simulink model "TAMC_PMSM"  (R2016b)
settings: Solver=ode15s  StartTime=0.0  StopTime=0.6  RelTol=1e-4
InitFcn:
  | Ts=10e-6;
  | R=0.958;
  | Ld=5.25e-3;
  | Lq=12e-3;
  | Pn=4;
  | flux=0.1827;
undefined symbols (not defined in the file or in its folder): DiscIntNeverNeededParam
libraries: powerlib x33, powerlib_extras x2
settings Model: Creator=ChenNingke  LastModifiedBy=CNK
settings SolverCC: MaxConsecutiveZCs=100000  ZeroCrossAlgorithm=Adaptive

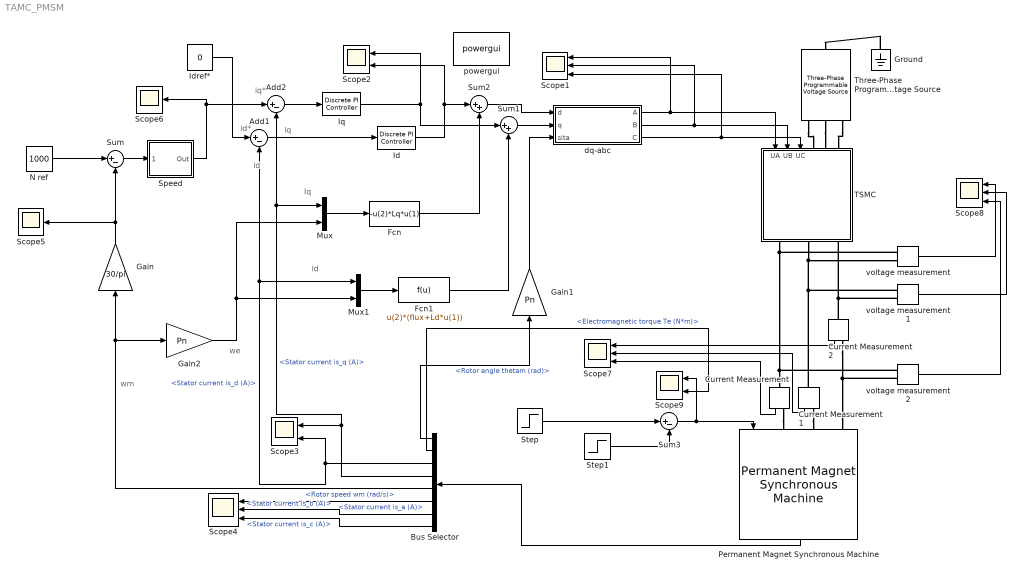
== system TAMC_PMSM ==
  note: we
  note: wm
  note: iq
  note: id
  note: id*
  note: iq*
  note: id
  note: Iq
  Add1 : Sum  Inputs=|+-
  Add2 : Sum  Inputs=|+-
  Bus Selector : BusSelector  OutputSignals=Rotor angle thetam (rad),Electromagnetic torque Te (N*m),Stator current is_d (A),Stator current is_q (A),Rotor speed wm (rad/s),Stator current is_a (A),Stator current is_b (A),Stator current is_c (A)
  Current Measurement : powerlib/Measurements/Current Measurement  PhasorSimulation=off  OutputType=Complex  PSBequivalent=0
  Current Measurement1 : powerlib/Measurements/Current Measurement  PhasorSimulation=off  OutputType=Complex  PSBequivalent=0
  Current Measurement2 : powerlib/Measurements/Current Measurement  PhasorSimulation=off  OutputType=Complex  PSBequivalent=0
  Fcn : Fcn  Expr=-u(2)*Lq*u(1)
  Fcn1 : Fcn  Expr=u(2)*(flux+Ld*u(1))
  Gain : Gain  Gain=30/pi
  Gain1 : Gain  Gain=Pn
  Gain2 : Gain  Gain=Pn
  Ground : powerlib/Elements/Ground  LConnTagsString=a
  Id : powerlib_extras/Discrete  Control Blocks/Discrete PI Controller  Kp=Ld*1100  Ki=R*1100  Par_Limits=[311*0.9*sqrt(1/3) -311*0.9*sqrt(1/3)]  Init=0  Ts=Ts
  Idref* : Constant  Value=0
  Iq : powerlib_extras/Discrete  Control Blocks/Discrete PI Controller  Kp=Lq*1100  Ki=R*1100  Par_Limits=[311*0.9*sqrt(1/3) -311*0.9*sqrt(1/3)]  Init=0  Ts=Ts
  Mux : Mux  Inputs=2
  Mux1 : Mux  Inputs=2
  "N ref " : Constant  Value=1000
  Permanent Magnet Synchronous Machine : powerlib/Machines/Permanent Magnet Synchronous Machine  NbPhases=3  FluxDistribution=Sinusoidal  RotorType=Salient-pole  MechanicalLoad=Torque Tm  PresetModel=No  ShowDetailedParameters=on  MeasurementBus=off  Resistance=0.958  Inductance=8.5e-3  dqInductances=[Ld,Lq]  La=0.000395  MachineConstant=Flux linkage established by magnets (V.s)  Flux=0.1827  VoltageCst=132.5525  TorqueCst=1.0962  Flat=120  Mechanical=[0.003 0 4 0]  PolePairs=4  InitialConditions=[0,0, 0,0]  InitialConditions5ph=[0 0 0 0 0 0]  TsPowergui=0  TsBlock=-1  RefAngle=90 degrees behind phase A axis (modified Park)
  Scope{1,4,7..8} (4 alike) : Scope  NumInputPorts=3
  Scope2 : Scope  NumInputPorts=2
  Scope3 : Scope  NumInputPorts=2
  Scope5 : Scope
  Scope6 : Scope
  Scope9 : Scope  NumInputPorts=2
  Speed : Subsystem  AncestorBlock=|  DialogController=POWERSYS.PowerSysDialog  mask(Discrete PI Controller){Kpw=0.14, Kiw=0.14*50, Ba=0.013, Par_Limits=[30 -30], Init=0, Ts=Ts}
      | powerlib_extras/Discrete 
      | Control Blocks/Discrete
      | PI Controller
      mask prompts: Kpw "Proportional gain (Kp):"; Kiw "Integral gain (Ki):"; Ba "feedback gain (Ba)"; Par_Limits "Output limits: [ Upper   Lower ]"; Init "Output initial value:"; Ts "Sample time:"
      mask help: This block implements a discrete PI controller.
      mask init:
      | UpperLimit=Par_Limits(1);
      | LowerLimit=Par_Limits(2);
      | power_initmask();
      mask Help: This block is part of a subset of blocks in the Extras library that does not have documentation associated with it, other than the block mask description.
      mask Display: disp('PI');
  Step : Step  Time=0.2  Before=1  After=10  SampleTime=Ts
  Step1 : Step  Time=0.4  After=3  SampleTime=Ts
  Sum : Sum  Inputs=|+-
  Sum1 : Sum  Inputs=|++
  Sum2 : Sum  Inputs=|++
  Sum3 : Sum  Inputs=|+-
  TSMC : Subsystem
  Three-Phase Programmable Voltage Source : powerlib/Electrical Sources/Three-Phase Programmable Voltage Source  PositiveSequence=[220 0 60]  VariationEntity=None  VariationType=Table of time-amplitude pairs  VariationTypeAlt=Step  VariationStep=0.5  VariationRate=10  VariationMagnitude=0.3  VariationFrequency=2  VariationTiming=[1 2]  VariationPhaseA=off  Amplitudes=[1 0.8 1.2 1.0]  TimeValues=[0 0.1 0.15 0.2]  HarmonicGeneration=off  HarmonicA=[3 0.2 -25 0]  HarmonicB=[2 0.15 35 2]  Timing="[0.05  3]"  BusType=swing  Pref=0  Qref=0  Qmin=-inf  Qmax=inf
  dq-abc : Subsystem
  powergui : powerlib/powergui  Priority=1  SimulationMode=Continuous  SolverType=Tustin/Backward Euler (TBE)  SampleTime=50e-6  frequency=60  SPID=off  DisableSnubberDevices=off  DisableRonSwitches=off  DisableVfSwitches=off  SwTol=0  DisplayEquations=off  Interpol=off  ExternalGateDelay=off  methode=off  Ts=10  FunctionMessages=off  echomessages=off  HookPort=off  EnableUseOfTLC=off  x0status=blocks  frequencyindice=0  Pbase=100e6  ErrMax=1e-4  Iterations=50  UnitsV=kV  UnitsW=MW  buscounter=0  RestoreLinks=warning  ResistiveCurrentMeasurement=off  Frange=[0:2:500]  Ylog=off  Xlog=on  ShowGrid=off  save=off  variable=ZData  structure=ScopeData6  ZoomFFT=off  StartTime=0.0  cycles=1  DisplayStyle=1  fundamental=60  FreqAxis=off  MaxFrequency=1000  frequencyindicesteady=1  RmsSteady=1  display=off
  voltage measurement : powerlib/Measurements/Voltage Measurement  PhasorSimulation=off  OutputType=Complex  PSBequivalent=0
  voltage measurement1 : powerlib/Measurements/Voltage Measurement  PhasorSimulation=off  OutputType=Complex  PSBequivalent=0
  voltage measurement2 : powerlib/Measurements/Voltage Measurement  PhasorSimulation=off  OutputType=Complex  PSBequivalent=0
  wires:
  dq-abc/1("A ") -> TSMC/1(UA), Scope1/1
  dq-abc/2("B ") -> TSMC/2(UB), Scope1/2
  Permanent Magnet Synchronous Machine/1 -> Bus Selector/1
  Bus Selector/5 -> Gain2/1, Gain/1  "<Rotor speed wm (rad/s)>"
  "N ref "/1 -> Sum/1
  Speed/1(Out) -> Add2/1, Scope6/1
  Id/1 -> Scope2/2, Sum2/1
  Iq/1 -> Sum1/1, Scope2/1
  Idref*/1 -> Add1/1
  Bus Selector/3 -> Mux1/1, Add1/2, Scope3/2  "<Stator current is_d (A)>"
  Bus Selector/4 -> Scope3/1, Mux/1, Add2/2  "<Stator current is_q (A)>"
  dq-abc/3("C ") -> TSMC/3(UC), Scope1/3
  Gain/1 -> Sum/2, Scope5/1
  Bus Selector/8 -> Scope4/3  "<Stator current is_c (A)>"
  Bus Selector/7 -> Scope4/2  "<Stator current is_b (A)>"
  Bus Selector/6 -> Scope4/1  "<Stator current is_a (A)>"
  Bus Selector/1 -> Gain1/1  "<Rotor angle thetam (rad)>"
  Sum/1 -> Speed/1(Error)
  Add2/1 -> Iq/1
  Add1/1 -> Id/1
  Sum2/1 -> dq-abc/1(d)
  Sum1/1 -> dq-abc/2(q)
  voltage measurement/1 -> Scope8/1
  voltage measurement1/1 -> Scope8/2
  voltage measurement2/1 -> Scope8/3
  Current Measurement/1 -> Scope7/3
  Current Measurement1/1 -> Scope7/2
  Current Measurement2/1 -> Scope7/1
  Gain1/1 -> dq-abc/3(sita)
  Mux/1 -> Fcn/1
  Mux1/1 -> Fcn1/1
  Gain2/1 -> Mux/2, Mux1/2
  Fcn/1 -> Sum2/2
  Fcn1/1 -> Sum1/2
  Step/1 -> Sum3/1
  Sum3/1 -> Permanent Magnet Synchronous Machine/1, Scope9/1
  Step1/1 -> Sum3/2
  Bus Selector/2 -> Scope9/2  "<Electromagnetic torque Te (N*m)>"
  connections:
  Three-Phase Programmable Voltage Source/RConn1 -- TSMC/LConn1
  Three-Phase Programmable Voltage Source/RConn2 -- TSMC/LConn2
  Three-Phase Programmable Voltage Source/RConn3 -- TSMC/LConn3
  Ground/LConn1 -- Three-Phase Programmable Voltage Source/LConn1
  TSMC/RConn1 -- voltage measurement/LConn1 -- voltage measurement2/LConn1 -- Current Measurement/LConn1
  Current Measurement1/LConn1 -- voltage measurement1/LConn1 -- voltage measurement/LConn2 -- TSMC/RConn2
  Current Measurement/RConn1 -- Permanent Magnet Synchronous Machine/LConn1
  Current Measurement1/RConn1 -- Permanent Magnet Synchronous Machine/LConn2
  Current Measurement2/RConn1 -- voltage measurement2/LConn2 -- Permanent Magnet Synchronous Machine/LConn3
  Current Measurement2/LConn1 -- TSMC/RConn3 -- voltage measurement1/LConn2

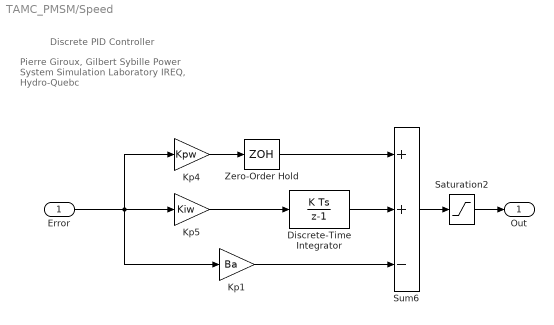
== system TAMC_PMSM/Speed ==
  note: Discrete PID Controller
  note: Pierre Giroux, Gilbert Sybille
      | Power System Simulation Laboratory
      | IREQ, Hydro-Quebc
  Error : Inport  SampleTime=Ts
  Discrete-Time Integrator : DiscreteIntegrator  InitialCondition=Init  SampleTime=Ts  LimitOutput=on  UpperSaturationLimit=UpperLimit  LowerSaturationLimit=LowerLimit  ICPrevOutput=DiscIntNeverNeededParam  ICPrevScaledInput=DiscIntNeverNeededParam
  Kp1 : Gain  Gain=Ba  SampleTime=Ts  SaturateOnIntegerOverflow=on  OutDataTypeStr=Inherit: Same as input  ParamDataTypeStr=Inherit: Same as input
  Kp4 : Gain  Gain=Kpw  SampleTime=Ts  SaturateOnIntegerOverflow=on  OutDataTypeStr=Inherit: Same as input  ParamDataTypeStr=Inherit: Same as input
  Kp5 : Gain  Gain=Kiw  SampleTime=Ts  SaturateOnIntegerOverflow=on  OutDataTypeStr=Inherit: Same as input  ParamDataTypeStr=Inherit: Same as input
  Saturation2 : Saturate  UpperLimit=UpperLimit  LowerLimit=LowerLimit  SampleTime=Ts
  Sum6 : Sum  Inputs=++-  SampleTime=Ts  SaturateOnIntegerOverflow=on  InputSameDT=on  OutDataTypeStr=Inherit: Same as first input
  Zero-Order Hold : ZeroOrderHold  SampleTime=Ts
  Out : Outport  SampleTime=Ts  InitialOutput=0
  wires:
  Error/1 -> Kp1/1, Kp5/1, Kp4/1
  Zero-Order Hold/1 -> Sum6/1
  Saturation2/1 -> Out/1
  Discrete-Time Integrator/1 -> Sum6/2
  Kp4/1 -> Zero-Order Hold/1
  Kp5/1 -> Discrete-Time Integrator/1
  Sum6/1 -> Saturation2/1
  Kp1/1 -> Sum6/3

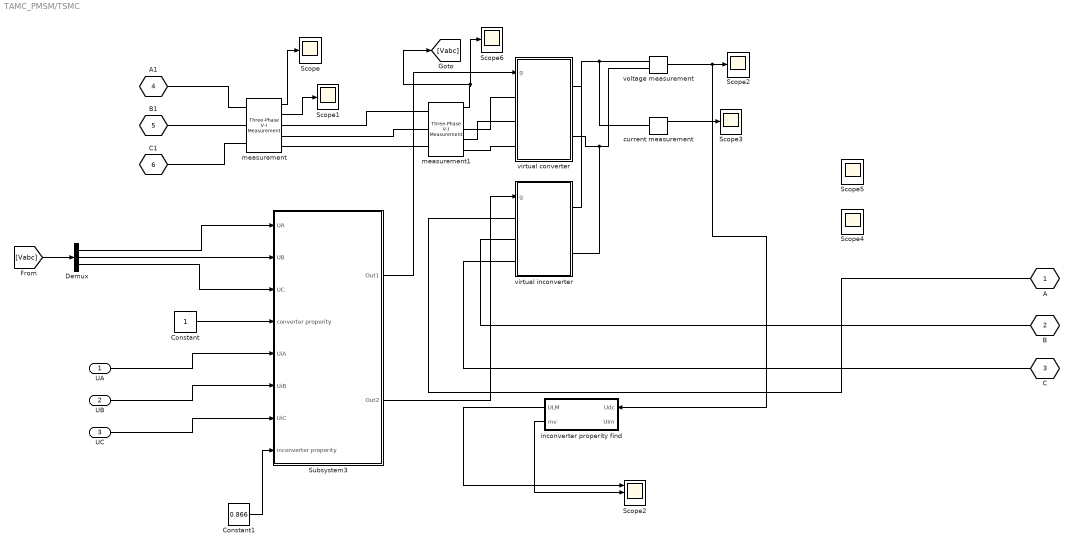
== system TAMC_PMSM/TSMC ==
  UA : Inport
  UB : Inport  Port=2
  UC : Inport  Port=3
  Constant : Constant
  Constant1 : Constant  Value=0.866
  Demux : Demux  Outputs=3
  Scope{,1,3..6} (6 alike) : Scope
  Scope2 : Scope  NumInputPorts=3
  "Scope2 " : Scope
  Subsystem3 : Subsystem
  current measurement : powerlib/Measurements/Current Measurement  PhasorSimulation=off  OutputType=Complex  PSBequivalent=0
  inconverter properity find : Subsystem
  measurement : powerlib/Measurements/Three-Phase V-I Measurement  VoltageMeasurement=phase-to-ground  SetLabelV=off  LabelV=Vabc  Vpu=off  VpuLL=off  CurrentMeasurement=yes  SetLabelI=off  LabelI=Iabc  Ipu=off  Pbase=100e6  Vbase=500e3  OutputType=Complex  PhasorSimulation=off  PSBequivalent=0
  measurement1 : powerlib/Measurements/Three-Phase V-I Measurement  VoltageMeasurement=phase-to-ground  SetLabelV=off  LabelV=Vabc  Vpu=off  VpuLL=off  CurrentMeasurement=yes  SetLabelI=off  LabelI=Iabc  Ipu=off  Pbase=100e6  Vbase=500e3  OutputType=Complex  PhasorSimulation=off  PSBequivalent=0
  virtual converter : Subsystem
  virtual inconverter : Subsystem
  voltage measurement : powerlib/Measurements/Voltage Measurement  PhasorSimulation=off  OutputType=Complex  PSBequivalent=0
  A : PMIOPort  Tag=PMCPort  Port=1  Side=Right
  B : PMIOPort  Tag=PMCPort  Port=2  Side=Right
  C : PMIOPort  Tag=PMCPort  Port=3  Side=Right
  A1 : PMIOPort  Tag=PMCPort  Port=4  Side=Left
  B1 : PMIOPort  Tag=PMCPort  Port=5  Side=Left
  C1 : PMIOPort  Tag=PMCPort  Port=6  Side=Left
  wires:
  voltage measurement/1 -> inconverter properity find/1(Udc), "Scope2 "/1
  current measurement/1 -> Scope3/1
  measurement/1 -> Scope/1
  Subsystem3/2(Out2) -> virtual inconverter/1(g)
  Subsystem3/1(Out1) -> virtual converter/1(g)
  measurement/2 -> Scope1/1
  Constant/1 -> Subsystem3/4(converter properity)
  inconverter properity find/1(ULM) -> Scope2/1
  inconverter properity find/2(mv) -> Scope2/2
  Constant1/1 -> Subsystem3/8(inconverter properity)
  Demux/1 -> Subsystem3/1(UA)
  Demux/2 -> Subsystem3/2(UB)
  Demux/3 -> Subsystem3/3(UC)
  UA/1 -> Subsystem3/5(UiA)
  UB/1 -> Subsystem3/6(UiB)
  UC/1 -> Subsystem3/7(UiC)
  measurement1/1 -> [Vabc], Scope6/1
  [Vabc] -> Demux/1
  connections:
  current measurement/LConn1 -- virtual inconverter/RConn1 -- virtual converter/RConn1 -- voltage measurement/LConn1
  virtual converter/RConn2 -- virtual inconverter/RConn2 -- voltage measurement/LConn2
  B1/RConn1 -- measurement/LConn2
  C1/RConn1 -- measurement/LConn3
  A1/RConn1 -- measurement/LConn1
  A/RConn1 -- virtual inconverter/LConn1
  B/RConn1 -- virtual inconverter/LConn2
  C/RConn1 -- virtual inconverter/LConn3
  measurement/RConn3 -- measurement1/LConn3
  measurement/RConn2 -- measurement1/LConn2
  measurement/RConn1 -- measurement1/LConn1
  measurement1/RConn1 -- virtual converter/LConn1
  measurement1/RConn2 -- virtual converter/LConn2
  measurement1/RConn3 -- virtual converter/LConn3

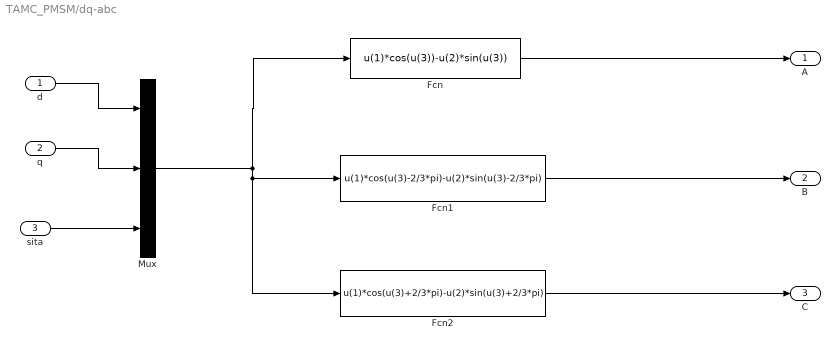
== system TAMC_PMSM/dq-abc ==
  d : Inport
  q : Inport  Port=2
  sita : Inport  Port=3
  Fcn : Fcn  Expr=u(1)*cos(u(3))-u(2)*sin(u(3))
  Fcn1 : Fcn  Expr=u(1)*cos(u(3)-2/3*pi)-u(2)*sin(u(3)-2/3*pi)
  Fcn2 : Fcn  Expr=u(1)*cos(u(3)+2/3*pi)-u(2)*sin(u(3)+2/3*pi)
  Mux : Mux  Inputs=3
  "A " : Outport
  "B " : Outport  Port=2
  "C " : Outport  Port=3
  wires:
  d/1 -> Mux/1
  q/1 -> Mux/2
  sita/1 -> Mux/3
  Fcn/1 -> "A "/1
  Fcn1/1 -> "B "/1
  Mux/1 -> Fcn/1, Fcn1/1, Fcn2/1
  Fcn2/1 -> "C "/1

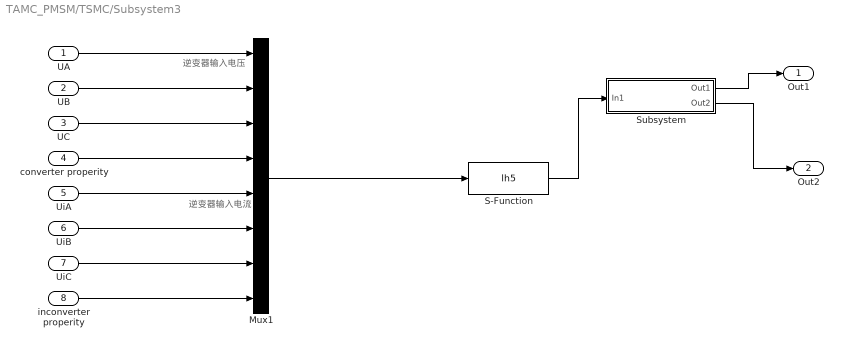
== system TAMC_PMSM/TSMC/Subsystem3 ==
  note: 逆变器输入电压
  note: 逆变器输入电流
  UA : Inport
  UB : Inport  Port=2
  UC : Inport  Port=3
  converter properity : Inport  Port=4
  UiA : Inport  Port=5
  UiB : Inport  Port=6
  UiC : Inport  Port=7
  inconverter properity : Inport  Port=8
  Mux1 : Mux  Inputs=8
  S-Function : S-Function  FunctionName=lh5  SFunctionDeploymentMode=off  EnableBusSupport=off
  Subsystem : Subsystem
  Out1 : Outport
  Out2 : Outport  Port=2
  wires:
  Subsystem/1(Out1) -> Out1/1
  S-Function/1 -> Subsystem/1(In1)
  Subsystem/2(Out2) -> Out2/1
  Mux1/1 -> S-Function/1
  UA/1 -> Mux1/1
  UB/1 -> Mux1/2
  UC/1 -> Mux1/3
  converter properity/1 -> Mux1/4
  inconverter properity/1 -> Mux1/8
  UiA/1 -> Mux1/5
  UiB/1 -> Mux1/6
  UiC/1 -> Mux1/7

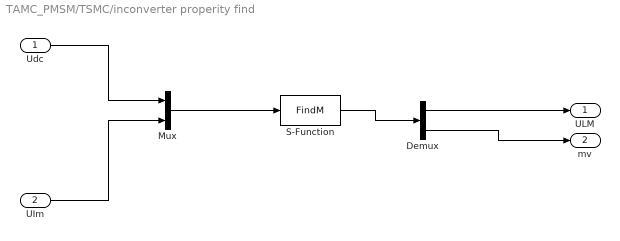
== system TAMC_PMSM/TSMC/inconverter properity find ==
  Udc : Inport
  UIm : Inport  Port=2
  Demux : Demux  Outputs=2
  Mux : Mux  Inputs=2
  S-Function : S-Function  FunctionName=FindM  SFunctionDeploymentMode=off  EnableBusSupport=off
  ULM : Outport
  mv : Outport  Port=2
  wires:
  Udc/1 -> Mux/1
  UIm/1 -> Mux/2
  Mux/1 -> S-Function/1
  S-Function/1 -> Demux/1
  Demux/1 -> ULM/1
  Demux/2 -> mv/1

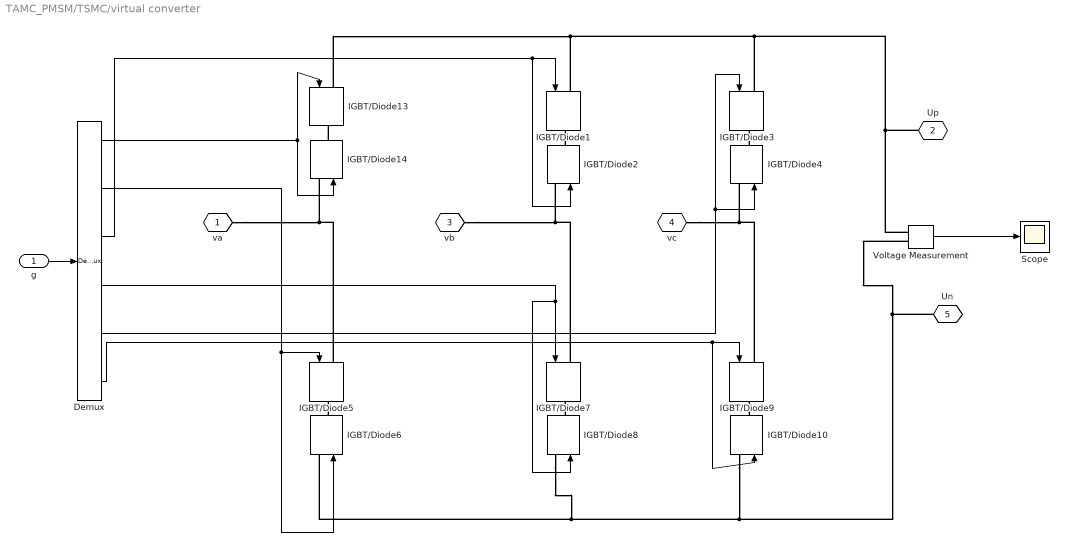
== system TAMC_PMSM/TSMC/virtual converter ==
  g : Inport
  Demux : Demux  Outputs=6
  IGBT/Diode{1..10,13..14} (12 alike) : powerlib/Power Electronics/IGBT//Diode  Ron=1e-3  Rs=1e5  Cs=inf  Measurements=off
  Scope : Scope
  Voltage Measurement : powerlib/Measurements/Voltage Measurement  PhasorSimulation=off  OutputType=Complex  PSBequivalent=0
  va : PMIOPort  Tag=PMCPort  Port=1  Side=Left
  Up : PMIOPort  Tag=PMCPort  Port=2  Side=Right
  vb : PMIOPort  Tag=PMCPort  Port=3  Side=Left
  vc : PMIOPort  Tag=PMCPort  Port=4  Side=Left
  Un : PMIOPort  Tag=PMCPort  Port=5  Side=Right
  wires:
  g/1 -> Demux/1
  Demux/1 -> IGBT/Diode13/1, IGBT/Diode14/1
  Demux/3 -> IGBT/Diode1/1, IGBT/Diode2/1
  Demux/5 -> IGBT/Diode4/1, IGBT/Diode3/1
  Voltage Measurement/1 -> Scope/1
  Demux/2 -> IGBT/Diode5/1, IGBT/Diode6/1
  Demux/4 -> IGBT/Diode8/1, IGBT/Diode7/1
  Demux/6 -> IGBT/Diode10/1, IGBT/Diode9/1
  connections:
  va/RConn1 -- IGBT/Diode5/LConn1 -- IGBT/Diode14/LConn1
  vb/RConn1 -- IGBT/Diode7/LConn1 -- IGBT/Diode2/LConn1
  vc/RConn1 -- IGBT/Diode9/LConn1 -- IGBT/Diode4/LConn1
  Up/RConn1 -- Voltage Measurement/LConn1 -- IGBT/Diode1/LConn1 -- IGBT/Diode13/LConn1 -- IGBT/Diode3/LConn1
  Voltage Measurement/LConn2 -- Un/RConn1 -- IGBT/Diode10/LConn1 -- IGBT/Diode6/LConn1 -- IGBT/Diode8/LConn1
  IGBT/Diode14/RConn1 -- IGBT/Diode13/RConn1
  IGBT/Diode2/RConn1 -- IGBT/Diode1/RConn1
  IGBT/Diode4/RConn1 -- IGBT/Diode3/RConn1
  IGBT/Diode6/RConn1 -- IGBT/Diode5/RConn1
  IGBT/Diode8/RConn1 -- IGBT/Diode7/RConn1
  IGBT/Diode10/RConn1 -- IGBT/Diode9/RConn1

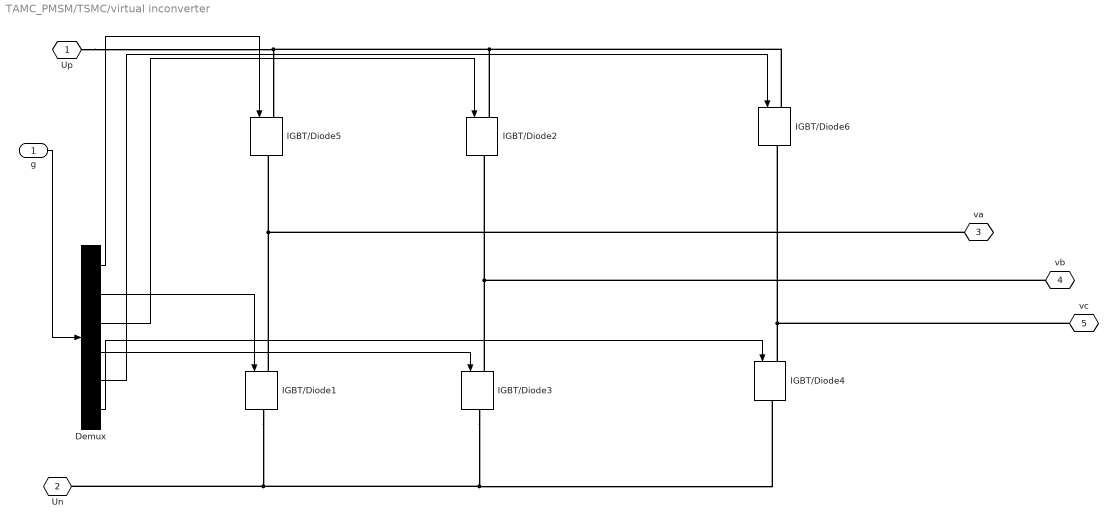
== system TAMC_PMSM/TSMC/virtual inconverter ==
  g : Inport
  Demux : Demux  Outputs=6
  IGBT/Diode{1..6} (6 alike) : powerlib/Power Electronics/IGBT//Diode  Ron=1e-3  Rs=1e5  Cs=inf  Measurements=off
  Up : PMIOPort  Tag=PMCPort  Port=1  Side=Right
  Un : PMIOPort  Tag=PMCPort  Port=2  Side=Right
  va : PMIOPort  Tag=PMCPort  Port=3  Side=Left
  vb : PMIOPort  Tag=PMCPort  Port=4  Side=Left
  vc : PMIOPort  Tag=PMCPort  Port=5  Side=Left
  wires:
  g/1 -> Demux/1
  Demux/1 -> IGBT/Diode5/1
  Demux/3 -> IGBT/Diode2/1
  Demux/5 -> IGBT/Diode6/1
  Demux/6 -> IGBT/Diode4/1
  Demux/2 -> IGBT/Diode1/1
  Demux/4 -> IGBT/Diode3/1
  connections:
  vc/RConn1 -- IGBT/Diode6/RConn1 -- IGBT/Diode4/LConn1
  vb/RConn1 -- IGBT/Diode2/RConn1 -- IGBT/Diode3/LConn1
  va/RConn1 -- IGBT/Diode1/LConn1 -- IGBT/Diode5/RConn1
  Up/RConn1 -- IGBT/Diode2/LConn1 -- IGBT/Diode6/LConn1 -- IGBT/Diode5/LConn1
  Un/RConn1 -- IGBT/Diode4/RConn1 -- IGBT/Diode3/RConn1 -- IGBT/Diode1/RConn1

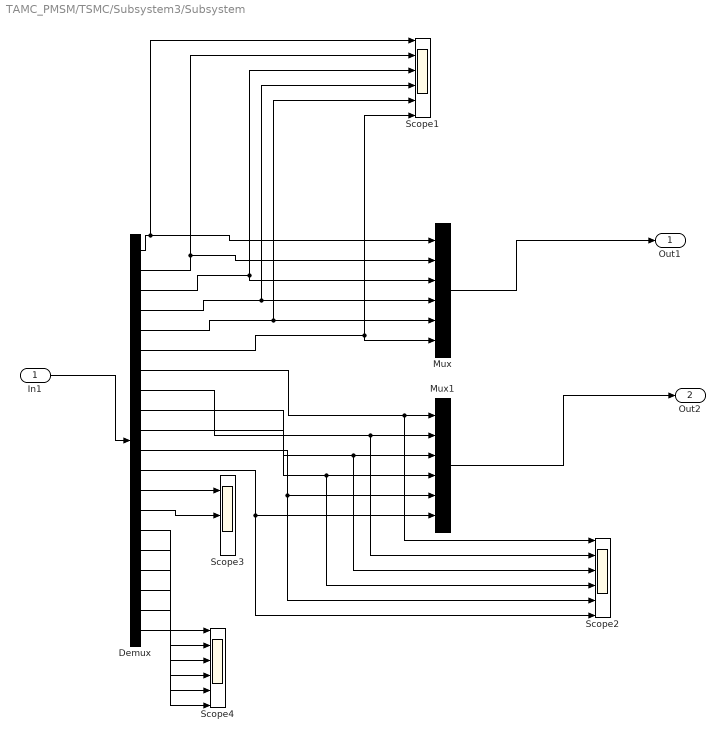
== system TAMC_PMSM/TSMC/Subsystem3/Subsystem ==
  In1 : Inport
  Demux : Demux  Outputs=20
  Mux : Mux  Inputs=6
  Mux1 : Mux  Inputs=6
  Scope1 : Scope  NumInputPorts=6
  Scope2 : Scope  NumInputPorts=6
  Scope3 : Scope  NumInputPorts=3
  Scope4 : Scope  NumInputPorts=6
  Out1 : Outport
  Out2 : Outport  Port=2
  wires:
  In1/1 -> Demux/1
  Demux/1 -> Mux/1, Scope1/1
  Demux/2 -> Mux/2, Scope1/2
  Demux/3 -> Mux/3, Scope1/3
  Demux/4 -> Scope1/4, Mux/4
  Demux/5 -> Scope1/5, Mux/5
  Mux/1 -> Out1/1
  Demux/6 -> Mux/6, Scope1/6
  Demux/7 -> Scope2/1, Mux1/1
  Demux/8 -> Scope2/2, Mux1/2
  Demux/9 -> Scope2/3, Mux1/3
  Demux/10 -> Scope2/4, Mux1/4
  Demux/11 -> Scope2/5, Mux1/5
  Demux/12 -> Scope2/6, Mux1/6
  Mux1/1 -> Out2/1
  Demux/13 -> Scope3/1
  Demux/14 -> Scope3/2
  Demux/15 -> Scope4/1
  Demux/16 -> Scope4/2
  Demux/17 -> Scope4/3
  Demux/18 -> Scope4/4
  Demux/19 -> Scope4/5
  Demux/20 -> Scope4/6
